simulink model "sampleModel2033"  (R2023a)
settings: Solver=VariableStepAuto  StartTime=0.0  StopTime=10.0  RelTol=1e-3
libraries: hdlsllib x11
settings Model: Creator=user1  LastModifiedBy=user1

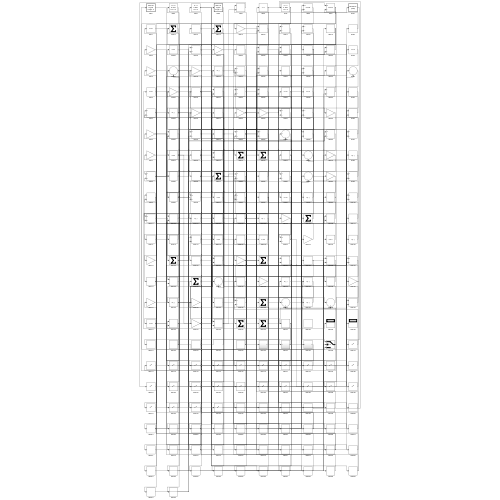
[thumbnail: Simulink's stored preview of the top-level diagram]
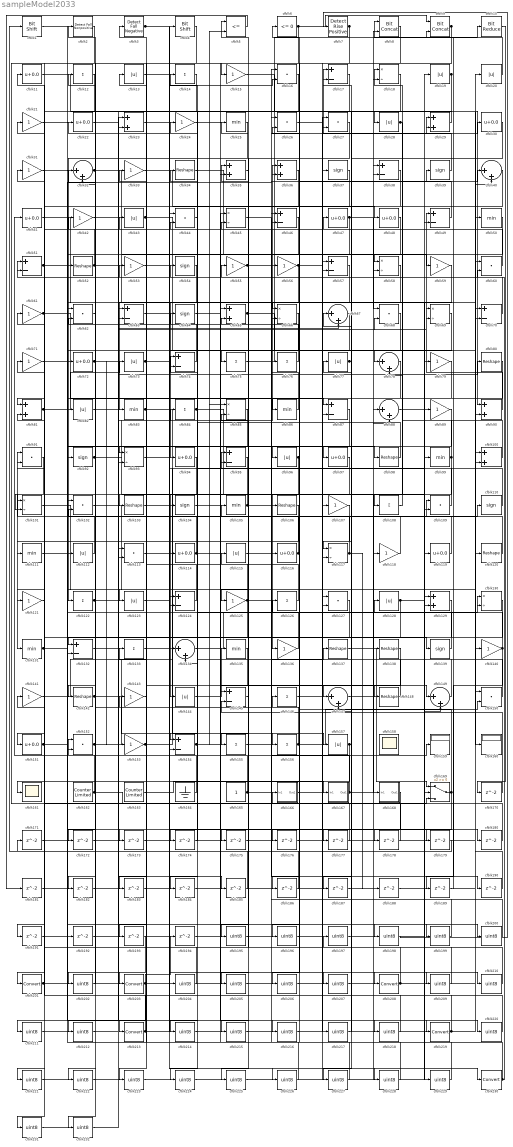
== system sampleModel2033 ==
  cfblk1 : hdlsllib/Logic and Bit Operations/Bit Shift  mode=Shift Left Logical  N=0
  cfblk10 : hdlsllib/Logic and Bit Operations/Bit Reduce  mode=AND
  cfblk{23,29,35..36,65,81,90,100,129} (9 alike) : Sum
  cfblk{18,45,58,66,69,85,93,101,117,130} (10 alike) : Product  Inputs=*/  RndMeth=Zero  SaturateOnIntegerOverflow=on
  cfblk{16,26..27,44,60,62,68,91,102,109,113,127,150,152} (14 alike) : DotProduct  OutDataTypeStr=Inherit: Inherit via internal rule
  cfblk{34,52,80,98,103,106,120,137..138,142,148} (11 alike) : Reshape
  cfblk{37,39,54,64,92,104,110,139} (8 alike) : Signum
  cfblk{25,50,83,86,99,105,111,131,135} (9 alike) : MinMax
  cfblk{15,21,24,31,33,42,53,55..56,59,61,71,79,89,107,118,121,125,136,140..141,143,153} (23 alike) : Gain
  cfblk{12,14,75..76,84,108,122,126,133,146,155..156} (12 alike) : Sum  Inputs=+
  cfblk{11,22,30,41,47..48,72,94,97,114,116,119,151} (13 alike) : Bias  Bias=0.0  SaturateOnIntegerOverflow=off
  cfblk{13,19..20,28,43,73,77,82,96,112,115,123,128,144,157} (15 alike) : Abs  SaturateOnIntegerOverflow=off
  cfblk{17,38,46,49,51,57,63,70,74,87,95,124,132,145,154} (15 alike) : Sum  Inputs=+-
  cfblk{32,40,67,78,88,134,147,149} (8 alike) : Sum  Inputs=|++
  cfblk158 : Scope
      settings: Floating=on
  cfblk159 : Display
  cfblk160 : Display
  cfblk161 : Scope
  cfblk162 : hdlsllib/Sources/Counter Limited  uplimit=7  tsamp=-1
  cfblk163 : hdlsllib/Sources/Counter Limited  uplimit=7  tsamp=-1
  cfblk164 : Ground
  cfblk165 : Constant  SampleTime=-1
  cfblk166 : Subsystem
      settings: LibrarySourceBlock=|
      | hdlsllib/Ports &
      | Subsystems/Subsystem
  cfblk167 : Subsystem
      settings: LibrarySourceBlock=|
      | hdlsllib/Ports &
      | Subsystems/Subsystem
  cfblk168 : Subsystem
      settings: LibrarySourceBlock=|
      | hdlsllib/Ports &
      | Subsystems/Subsystem
  cfblk169 : Switch  SaturateOnIntegerOverflow=off  InputSameDT=off
  cfblk{170..194} (25 alike) : Delay  SampleTime=1
  cfblk{195..200,202,204..207,209..212,214..218,220..229,231..232} (32 alike) : DataTypeConversion  OutDataTypeStr=uint8  SaturateOnIntegerOverflow=off  RndMeth=Floor
  cfblk2 : hdlsllib/Logic and Bit Operations/Detect Fall Nonpositive  vinit=0  OutDataTypeStr=boolean
  cfblk{201,203,208,213,219,230} (6 alike) : DataTypeConversion  SaturateOnIntegerOverflow=off  RndMeth=Floor
  cfblk3 : hdlsllib/Logic and Bit Operations/Detect Fall Negative  vinit=0  OutDataTypeStr=boolean
  cfblk4 : hdlsllib/Logic and Bit Operations/Bit Shift  mode=Shift Left Logical  N=0
  cfblk5 : RelationalOperator  Operator=<=  OutDataTypeStr=boolean  InputSameDT=off
  cfblk6 : hdlsllib/Logic and Bit Operations/Compare To Zero  relop=<=  OutDataTypeStr=boolean
  cfblk7 : hdlsllib/Logic and Bit Operations/Detect Rise Positive  vinit=0  OutDataTypeStr=boolean
  cfblk8 : hdlsllib/Logic and Bit Operations/Bit Concat  numInputs=2
  cfblk9 : hdlsllib/Logic and Bit Operations/Bit Concat  numInputs=2
  wires:
  cfblk25/1 -> cfblk122/1
  cfblk11/1 -> cfblk90/1
  cfblk39/1 -> cfblk17/1
  cfblk141/1 -> cfblk110/1
  cfblk116/1 -> cfblk91/1, cfblk5/1
  cfblk43/1 -> cfblk75/1, cfblk109/2, cfblk193/1
  cfblk57/1 -> cfblk125/1
  cfblk65/1 -> cfblk10/1, cfblk100/2
  cfblk143/1 -> cfblk203/1
  cfblk131/1 -> cfblk109/1, cfblk176/1
  cfblk83/1 -> cfblk156/1, cfblk43/1
  cfblk54/1 -> cfblk83/1
  cfblk48/1 -> cfblk132/1
  cfblk56/1 -> cfblk58/1, cfblk134/2
  cfblk6/1 -> cfblk9/1, cfblk121/1
  cfblk153/1 -> cfblk128/1, cfblk130/2
  cfblk96/1 -> cfblk144/1, cfblk101/2
  cfblk80/1 -> cfblk102/1
  cfblk59/1 -> cfblk94/1
  cfblk137/1 -> cfblk169/1
  cfblk97/1 -> cfblk136/1
  cfblk29/1 -> cfblk28/1
  cfblk108/1 -> cfblk18/1
  cfblk134/1 -> cfblk18/2
  cfblk81/1 -> cfblk73/1, cfblk36/2, cfblk139/1
  cfblk114/1 -> cfblk32/1, cfblk148/1
  cfblk75/1 -> cfblk29/1
  cfblk42/1 -> cfblk140/1
  cfblk164/1 -> cfblk41/1
  cfblk49/1 -> cfblk6/1
  cfblk100/1 -> cfblk54/1
  cfblk72/1 -> cfblk87/1, cfblk153/1
  cfblk92/1 -> cfblk36/1, cfblk117/2
  cfblk144/1 -> cfblk135/1
  cfblk2/1 -> cfblk166/1(In1)
  cfblk61/1 -> cfblk86/1, cfblk98/1
  cfblk68/1 -> cfblk72/1
  cfblk31/1 -> cfblk123/1
  cfblk33/1 -> cfblk48/1
  cfblk155/1 -> cfblk137/1
  cfblk13/1 -> cfblk208/1
  cfblk90/1 -> cfblk49/1
  cfblk150/1 -> cfblk51/1
  cfblk156/1 -> cfblk150/2, cfblk32/2
  cfblk47/1 -> cfblk68/1, cfblk74/2
  cfblk74/1 -> cfblk2/1
  cfblk1/1 -> cfblk82/1
  cfblk41/1 -> cfblk116/1
  cfblk154/1 -> cfblk5/2, cfblk180/1
  cfblk19/1 -> cfblk142/1, cfblk147/2, cfblk93/2
  cfblk119/1 -> cfblk105/1
  cfblk79/1 -> cfblk97/1
  cfblk121/1 -> cfblk71/1
  cfblk102/1 -> cfblk168/1(In1)
  cfblk124/1 -> cfblk3/1
  cfblk69/1 -> cfblk154/1
  cfblk14/1 -> cfblk81/1
  cfblk125/1 -> cfblk64/1, cfblk39/1, cfblk30/1, cfblk149/1, cfblk174/1
  cfblk99/1 -> cfblk131/1, cfblk45/2
  cfblk30/1 -> cfblk117/1
  cfblk84/1 -> cfblk138/1, cfblk85/1
  cfblk136/1 -> cfblk34/1
  cfblk117/1 -> cfblk61/1, cfblk188/1
  cfblk147/1 -> cfblk118/1
  cfblk142/1 -> cfblk89/1, cfblk68/2, cfblk204/1
  cfblk105/1 -> cfblk103/1, cfblk40/1, cfblk69/2
  cfblk52/1 -> cfblk119/1, cfblk67/2, cfblk42/1
  cfblk162/1 -> cfblk152/1, cfblk169/3
  cfblk85/1 -> cfblk132/2
  cfblk20/1 -> cfblk8/1
  cfblk106/1 -> cfblk151/1
  cfblk77/1 -> cfblk147/1, cfblk187/1
  cfblk67/1 -> cfblk92/1
  cfblk15/1 -> cfblk120/1
  cfblk152/1 -> cfblk20/1, cfblk232/1
  cfblk112/1 -> cfblk31/1
  cfblk89/1 -> cfblk154/2
  cfblk98/1 -> cfblk24/1
  cfblk148/1 -> cfblk55/1
  cfblk93/1 -> cfblk16/2
  cfblk101/1 -> cfblk160/1
  cfblk86/1 -> cfblk76/1
  cfblk87/1 -> cfblk96/1
  cfblk40/1 -> cfblk111/1
  cfblk82/1 -> cfblk80/1
  cfblk91/1 -> cfblk101/1
  cfblk149/1 -> cfblk22/1
  cfblk126/1 -> cfblk25/1
  cfblk4/1 -> cfblk52/1
  cfblk123/1 -> cfblk95/1
  cfblk3/1 -> cfblk78/1, cfblk226/1
  cfblk55/1 -> cfblk106/1, cfblk157/1
  cfblk109/1 -> cfblk56/1
  cfblk66/1 -> cfblk95/2
  cfblk107/1 -> cfblk127/2
  cfblk110/1 -> cfblk14/1
  cfblk73/1 -> cfblk4/1, cfblk93/1
  cfblk9/1 -> cfblk57/2, cfblk223/1
  cfblk151/1 -> cfblk130/1, cfblk200/1
  cfblk17/1 -> cfblk114/1
  cfblk140/1 -> cfblk67/1, cfblk189/1
  cfblk94/1 -> cfblk124/2
  cfblk113/1 -> cfblk219/1
  cfblk35/1 -> cfblk155/1
  cfblk165/1 -> cfblk74/1, cfblk159/1
  cfblk104/1 -> cfblk145/1
  cfblk70/1 -> cfblk11/1
  cfblk78/1 -> cfblk112/1
  cfblk120/1 -> cfblk77/1
  cfblk7/1 -> cfblk15/1, cfblk196/1
  cfblk122/1 -> cfblk84/1, cfblk69/1
  cfblk76/1 -> cfblk53/1
  cfblk50/1 -> cfblk213/1
  cfblk60/1 -> cfblk21/1
  cfblk145/1 -> cfblk65/2
  cfblk34/1 -> cfblk107/1
  cfblk169/1 -> cfblk126/1, cfblk224/1
  cfblk32/1 -> cfblk59/1, cfblk66/2
  cfblk139/1 -> cfblk115/1
  cfblk167/1(Out1) -> cfblk35/1, cfblk29/2
  cfblk28/1 -> cfblk108/1, cfblk78/2
  cfblk51/1 -> cfblk70/2, cfblk161/1
  cfblk118/1 -> cfblk33/1
  cfblk8/1 -> cfblk35/2
  cfblk157/1 -> cfblk191/1, cfblk227/1
  cfblk128/1 -> cfblk149/2, cfblk184/1
  cfblk44/1 -> cfblk104/1
  cfblk163/1 -> cfblk167/1(In1)
  cfblk53/1 -> cfblk66/1
  cfblk12/1 -> cfblk201/1
  cfblk63/1 -> cfblk230/1
  cfblk10/1 -> cfblk170/1
  cfblk170/1 -> cfblk145/2
  cfblk171/1 -> cfblk127/1
  cfblk16/1 -> cfblk172/1
  cfblk172/1 -> cfblk65/1
  cfblk111/1 -> cfblk173/1
  cfblk173/1 -> cfblk100/1
  cfblk174/1 -> cfblk44/2
  cfblk58/1 -> cfblk175/1
  cfblk175/1 -> cfblk88/1
  cfblk176/1 -> cfblk60/1
  cfblk18/1 -> cfblk177/1
  cfblk177/1 -> cfblk51/2
  cfblk45/1 -> cfblk178/1
  cfblk178/1 -> cfblk62/2
  cfblk103/1 -> cfblk179/1
  cfblk179/1 -> cfblk1/1
  cfblk180/1 -> cfblk17/2
  cfblk5/1 -> cfblk181/1
  cfblk181/1 -> cfblk57/1
  cfblk36/1 -> cfblk182/1
  cfblk182/1 -> cfblk150/1
  cfblk135/1 -> cfblk183/1
  cfblk183/1 -> cfblk8/2
  cfblk22/1 -> cfblk185/1
  cfblk185/1 -> cfblk81/2
  cfblk130/1 -> cfblk186/1
  cfblk186/1 -> cfblk124/1
  cfblk187/1 -> cfblk90/2
  cfblk188/1 -> cfblk169/2
  cfblk189/1 -> cfblk9/2
  cfblk115/1 -> cfblk190/1
  cfblk190/1 -> cfblk70/1
  cfblk191/1 -> cfblk49/2
  cfblk71/1 -> cfblk192/1
  cfblk192/1 -> cfblk102/2
  cfblk194/1 -> cfblk19/1
  cfblk27/1 -> cfblk195/1
  cfblk195/1 -> cfblk99/1
  cfblk196/1 -> cfblk27/1
  cfblk197/1 -> cfblk27/2
  cfblk26/1 -> cfblk198/1
  cfblk198/1 -> cfblk7/1
  cfblk166/1(Out1) -> cfblk199/1
  cfblk199/1 -> cfblk26/1
  cfblk200/1 -> cfblk26/2
  cfblk201/1 -> cfblk152/2, cfblk58/2
  cfblk62/1 -> cfblk202/1
  cfblk202/1 -> cfblk12/1
  cfblk203/1 -> cfblk194/1, cfblk221/1
  cfblk204/1 -> cfblk143/1
  cfblk38/1 -> cfblk205/1
  cfblk205/1 -> cfblk79/1
  cfblk168/1(Out1) -> cfblk206/1
  cfblk206/1 -> cfblk38/1
  cfblk184/1 -> cfblk207/1
  cfblk207/1 -> cfblk38/2
  cfblk208/1 -> cfblk171/1, cfblk40/2, cfblk85/2
  cfblk64/1 -> cfblk209/1
  cfblk209/1 -> cfblk13/1
  cfblk23/1 -> cfblk210/1
  cfblk210/1 -> cfblk44/1
  cfblk127/1 -> cfblk211/1
  cfblk211/1 -> cfblk23/1
  cfblk193/1 -> cfblk212/1
  cfblk212/1 -> cfblk23/2
  cfblk213/1 -> cfblk134/1, cfblk141/1
  cfblk138/1 -> cfblk214/1
  cfblk214/1 -> cfblk50/1
  cfblk37/1 -> cfblk215/1
  cfblk215/1 -> cfblk16/1
  cfblk132/1 -> cfblk216/1
  cfblk216/1 -> cfblk37/1
  cfblk146/1 -> cfblk217/1
  cfblk217/1 -> cfblk47/1
  cfblk24/1 -> cfblk218/1
  cfblk218/1 -> cfblk146/1
  cfblk219/1 -> cfblk197/1, cfblk91/2
  cfblk21/1 -> cfblk220/1
  cfblk220/1 -> cfblk113/1
  cfblk221/1 -> cfblk113/2
  cfblk129/1 -> cfblk222/1
  cfblk222/1 -> cfblk87/2
  cfblk223/1 -> cfblk129/1
  cfblk224/1 -> cfblk129/2
  cfblk46/1 -> cfblk225/1
  cfblk225/1 -> cfblk88/2
  cfblk226/1 -> cfblk46/1
  cfblk227/1 -> cfblk46/2
  cfblk133/1 -> cfblk228/1
  cfblk228/1 -> cfblk62/1
  cfblk88/1 -> cfblk229/1
  cfblk229/1 -> cfblk133/1
  cfblk230/1 -> cfblk45/1, cfblk60/2
  cfblk95/1 -> cfblk231/1
  cfblk231/1 -> cfblk63/1
  cfblk232/1 -> cfblk63/2

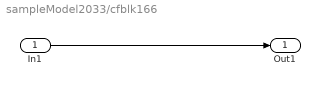
== system sampleModel2033/cfblk166 ==
  In1 : Inport
  Out1 : Outport
  wires:
  In1/1 -> Out1/1

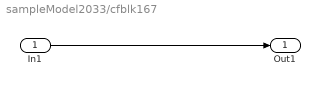
== system sampleModel2033/cfblk167 ==
  In1 : Inport
  Out1 : Outport
  wires:
  In1/1 -> Out1/1

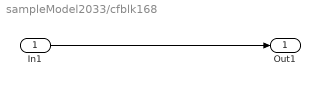
== system sampleModel2033/cfblk168 ==
  In1 : Inport
  Out1 : Outport
  wires:
  In1/1 -> Out1/1
